simulink model "Pend_model"  (R2020b)
settings: Solver=VariableStepAuto  StartTime=0.0  StopTime=5  RelTol=1e-3
values from neighbouring files (symbols this model uses):
  A = eval(Ar)    [Script_pendul.m]    (also in extended_kalman_filter.m = I+Ts*eval(subs(jac,[x_sym,u_sym]',[x_est(:,k);u(:,k)])))
  B = eval(Br)    [Script_pendul.m]
  C = [1 0 0 0;0 0 1 0]    [Script_pendul.m]    (also in extended_kalman_filter.m = eval(subs(out_jac,x_sym',x_pred)))
  K = place(A,B,poles)    [Script_pendul.m]
  L = L'    [Script_pendul.m]
settings Model: Creator=tudor  LastModifiedBy=tudor

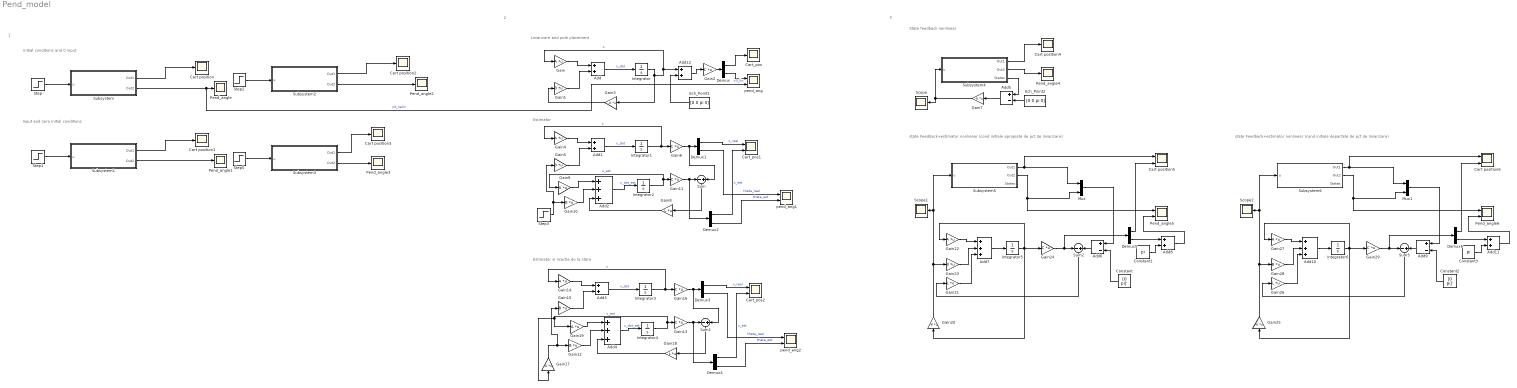
== system Pend_model ==
  note: 3
  note: State feedback nonlinear
  note: 2
  note: Estimator
  note: Liniarizare and pole placement
  note: 1
  note: Input and zero initial conditions
  note: Initial conditions and 0 input
  note: Estimator si reactie de la stare
  note: state Feedback+estimator nonlinear (cond initiale apropiate de pct de liniarizare)
  note: state Feedback+estimator nonlinear (cond initiale departate de pct de liniarizare)
  Add{,1,3,8,11..12} (6 alike) : Sum
  Add{2,4,7,10} (4 alike) : Sum  Inputs=+++
  Add5 : Sum  Inputs=+-
  Add6 : Sum  Inputs=+-
  Add9 : Sum  Inputs=+-
  Cart position{,1..4} (5 alike) : Scope
  Cart position5 : Scope  NumInputPorts=2
  Cart position6 : Scope  NumInputPorts=2
  Cart_pos : Scope
  Cart_pos1 : Scope  NumInputPorts=2
  Cart_pos2 : Scope  NumInputPorts=2
  Constant : Constant  Value=[0 pi]'
  Constant1 : Constant  Value=pi
  Constant2 : Constant  Value=[0 pi]'
  Constant3 : Constant  Value=pi
  Demux{,1..6} (7 alike) : Demux  Outputs=2
  Ech_Point1 : Constant  Value=[0 0 pi 0]
  Ech_Point2 : Constant  Value=[0 0 pi 0]
  Gain{,4,9,14,19,22,27} (7 alike) : Gain  Gain=A  Multiplication=Matrix(K*u)
  Gain{1,5,10,12,15,23,28} (7 alike) : Gain  Gain=B  Multiplication=Matrix(K*u)
  Gain{2,6,11,13,16,24,29} (7 alike) : Gain  Gain=C  Multiplication=Matrix(K*u)
  Gain{3,7,17,20,25} (5 alike) : Gain  Gain=-K  Multiplication=Matrix(K*u)
  Gain{8,18,21,26} (4 alike) : Gain  Gain=L  Multiplication=Matrix(K*u)
  Integrator : Integrator  InitialCondition=[0 0 0.01 0]
  Integrator1 : Integrator  InitialCondition=[0 0 0.1 0]
  Integrator2 : Integrator  InitialCondition=[0 0 0.5 0]
  Integrator3 : Integrator  InitialCondition=[0 0 0.1 0]
  Integrator4 : Integrator  InitialCondition=[0 0 1 0]
  Integrator5 : Integrator  InitialCondition=[0 0 0.5 0]
  Integrator6 : Integrator  InitialCondition=[0 0 0.5 0]
  Mux : Mux  Inputs=2
  Mux1 : Mux  Inputs=2
  Pend_angle{,1..4} (5 alike) : Scope
  Pend_angle5 : Scope  NumInputPorts=2
  Pend_angle6 : Scope  NumInputPorts=2
  Scope : Scope
  Scope1 : Scope
  Scope2 : Scope
  Step : Step  Time=0  After=0  SampleTime=0
  Step1 : Step  Before=10  After=0  SampleTime=0
  Step2 : Step  Time=0  After=0  SampleTime=0
  Step3 : Step  Time=0  After=0  SampleTime=0
  Step5 : Step  Before=0.1  After=0  SampleTime=0
  Subsystem : Subsystem
  Subsystem1 : Subsystem
  Subsystem2 : Subsystem
  Subsystem3 : Subsystem
  Subsystem4 : Subsystem
  Subsystem5 : Subsystem
  Subsystem6 : Subsystem
  Sum{,1..3} (4 alike) : Sum  Inputs=-|+
  pend_ang : Scope  NumInputPorts=2
  pend_ang1 : Scope  NumInputPorts=2
  pend_ang2 : Scope  NumInputPorts=2
  wires:
  Step/1 -> Subsystem/1(u)
  Subsystem/1(Out1) -> Cart position/1
  Subsystem/2(Out2) -> pend_ang/2, Pend_angle/1  "x3_nelin"
  Step1/1 -> Subsystem1/1(u)
  Subsystem1/2(Out2) -> Pend_angle1/1
  Subsystem1/1(Out1) -> Cart position1/1
  Step2/1 -> Subsystem2/1(u)
  Subsystem2/2(Out2) -> Pend_angle2/1
  Subsystem2/1(Out1) -> Cart position2/1
  Subsystem3/2(Out2) -> Pend_angle3/1
  Step5/1 -> Subsystem3/1(u)
  Subsystem3/1(Out1) -> Cart position3/1
  Gain/1 -> Add/1
  Gain1/1 -> Add/2
  Add/1 -> Integrator/1  "x_dot"
  Integrator/1 -> Gain3/1, Add12/1, Gain/1  "x"
  Gain3/1 -> Gain1/1
  Gain2/1 -> Demux/1
  Demux/1 -> Cart_pos/1
  Demux/2 -> pend_ang/1  "x3_lin"
  Gain6/1 -> Sum/2, Demux1/1
  Add1/1 -> Integrator1/1  "x_dot"
  Integrator1/1 -> Gain6/1, Gain4/1  "x"
  Gain5/1 -> Add1/2
  Demux1/2 -> pend_ang1/1  "theta_real"
  Gain4/1 -> Add1/1
  Demux1/1 -> Cart_pos1/1  "x_real"
  Sum/1 -> Gain8/1
  Gain8/1 -> Add2/3
  Add2/1 -> Integrator2/1  "x_dot_est"
  Integrator2/1 -> Gain9/1, Gain11/1  "x_est"
  Gain10/1 -> Add2/2
  Gain9/1 -> Add2/1
  Step3/1 -> Gain5/1, Gain10/1
  Gain11/1 -> Demux2/1, Sum/1
  Demux2/1 -> Cart_pos1/2  "x_est"
  Demux2/2 -> pend_ang1/2  "theta_est"
  Demux4/2 -> pend_ang2/2  "theta_est"
  Demux3/1 -> Cart_pos2/1  "x_real"
  Add3/1 -> Integrator3/1  "x_dot"
  Gain15/1 -> Add3/2
  Integrator3/1 -> Gain16/1, Gain14/1  "x"
  Gain16/1 -> Sum1/2, Demux3/1
  Gain13/1 -> Demux4/1, Sum1/1
  Integrator4/1 -> Gain17/1, Gain19/1, Gain13/1  "x_est"
  Demux3/2 -> pend_ang2/1  "theta_real"
  Gain17/1 -> Gain15/1, Gain12/1
  Demux4/1 -> Cart_pos2/2  "x_est"
  Gain18/1 -> Add4/3
  Sum1/1 -> Gain18/1
  Gain19/1 -> Add4/1
  Add4/1 -> Integrator4/1  "x_dot_est"
  Gain14/1 -> Add3/1
  Gain12/1 -> Add4/2
  Subsystem4/1(Out1) -> Cart position4/1
  Subsystem4/2(Out2) -> Pend_angle4/1
  Ech_Point2/1 -> Add5/2
  Gain7/1 -> Scope/1, Subsystem4/1(u)
  Subsystem4/3(States) -> Add5/1
  Add5/1 -> Gain7/1
  Subsystem5/2(Out2) -> Mux/2, Pend_angle5/1
  Subsystem5/1(Out1) -> Mux/1, Cart position5/1
  Sum2/1 -> Gain21/1
  Gain22/1 -> Add7/1
  Gain23/1 -> Add7/2
  Gain21/1 -> Add7/3
  Add7/1 -> Integrator5/1
  Demux5/1 -> Cart position5/2
  Gain24/1 -> Demux5/1, Sum2/1
  Integrator5/1 -> Gain22/1, Gain24/1, Gain20/1
  Gain20/1 -> Subsystem5/1(u), Scope1/1, Gain23/1
  Mux/1 -> Add6/1
  Add6/1 -> Sum2/2
  Constant/1 -> Add6/2
  Constant1/1 -> Add8/2
  Demux5/2 -> Add8/1
  Add8/1 -> Pend_angle5/2
  Subsystem6/2(Out2) -> Mux1/2, Pend_angle6/1
  Gain25/1 -> Subsystem6/1(u), Scope2/1, Gain28/1
  Subsystem6/1(Out1) -> Mux1/1, Cart position6/1
  Gain26/1 -> Add10/3
  Add10/1 -> Integrator6/1
  Integrator6/1 -> Gain27/1, Gain29/1, Gain25/1
  Demux6/1 -> Cart position6/2
  Gain28/1 -> Add10/2
  Constant3/1 -> Add11/2
  Sum3/1 -> Gain26/1
  Gain29/1 -> Demux6/1, Sum3/1
  Constant2/1 -> Add9/2
  Mux1/1 -> Add9/1
  Gain27/1 -> Add10/1
  Demux6/2 -> Add11/1
  Add9/1 -> Sum3/2
  Add11/1 -> Pend_angle6/2
  Ech_Point1/1 -> Add12/2
  Add12/1 -> Gain2/1

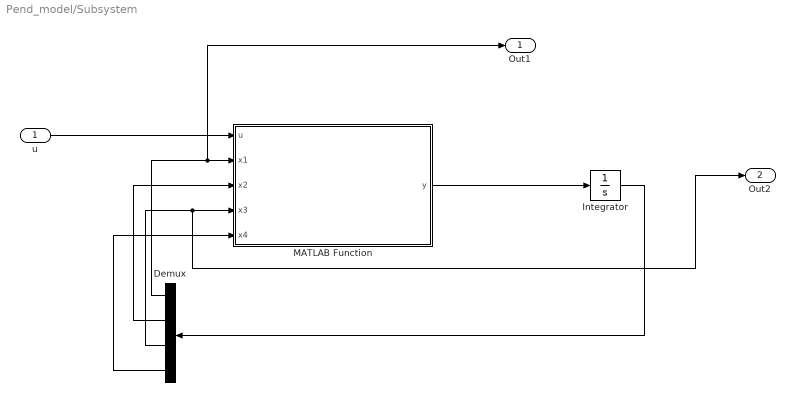
== system Pend_model/Subsystem ==
  u : Inport
  Demux : Demux
  Integrator : Integrator  InitialCondition=[0 0 pi+0.01 0]
  MATLAB Function : MATLAB Function  TreatAsAtomicUnit=on
  Out1 : Outport
  Out2 : Outport  Port=2
  wires:
  Integrator/1 -> Demux/1
  Demux/4 -> MATLAB Function/5(x4)
  MATLAB Function/1(y) -> Integrator/1
  Demux/3 -> Out2/1, MATLAB Function/4(x3)
  Demux/1 -> Out1/1, MATLAB Function/2(x1)
  Demux/2 -> MATLAB Function/3(x2)
  u/1 -> MATLAB Function/1(u)

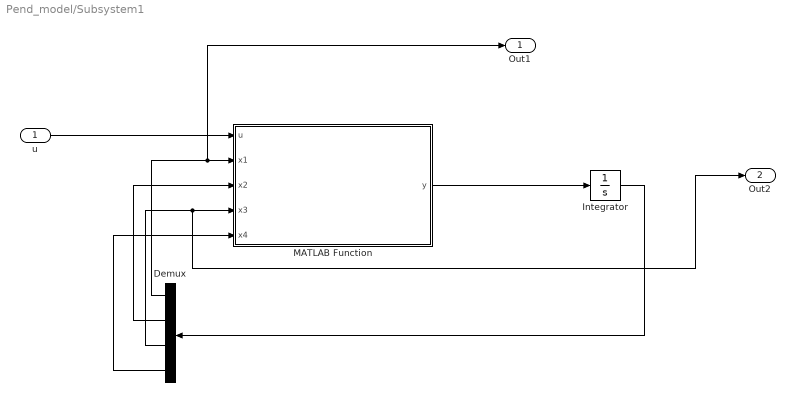
== system Pend_model/Subsystem1 ==
  u : Inport
  Demux : Demux
  Integrator : Integrator  InitialCondition=[0 0 0 0]
  MATLAB Function : MATLAB Function  TreatAsAtomicUnit=on
  Out1 : Outport
  Out2 : Outport  Port=2
  wires:
  Integrator/1 -> Demux/1
  Demux/4 -> MATLAB Function/5(x4)
  MATLAB Function/1(y) -> Integrator/1
  Demux/3 -> Out2/1, MATLAB Function/4(x3)
  Demux/1 -> Out1/1, MATLAB Function/2(x1)
  Demux/2 -> MATLAB Function/3(x2)
  u/1 -> MATLAB Function/1(u)

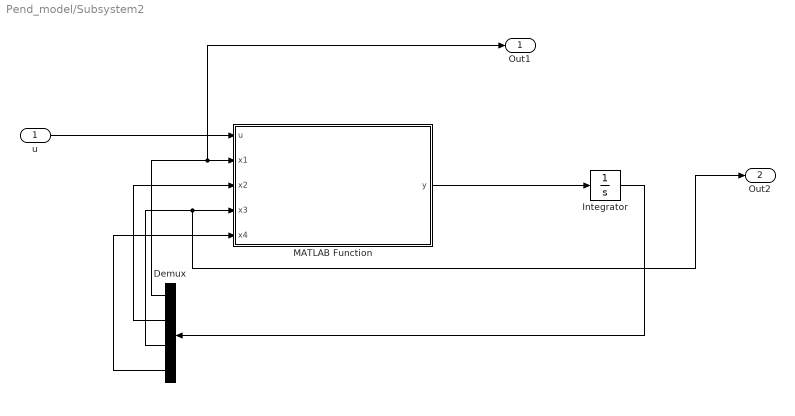
== system Pend_model/Subsystem2 ==
  u : Inport
  Demux : Demux
  Integrator : Integrator  InitialCondition=[0 0 pi 0]
  MATLAB Function : MATLAB Function  TreatAsAtomicUnit=on
  Out1 : Outport
  Out2 : Outport  Port=2
  wires:
  Integrator/1 -> Demux/1
  Demux/4 -> MATLAB Function/5(x4)
  MATLAB Function/1(y) -> Integrator/1
  Demux/3 -> Out2/1, MATLAB Function/4(x3)
  Demux/1 -> Out1/1, MATLAB Function/2(x1)
  Demux/2 -> MATLAB Function/3(x2)
  u/1 -> MATLAB Function/1(u)

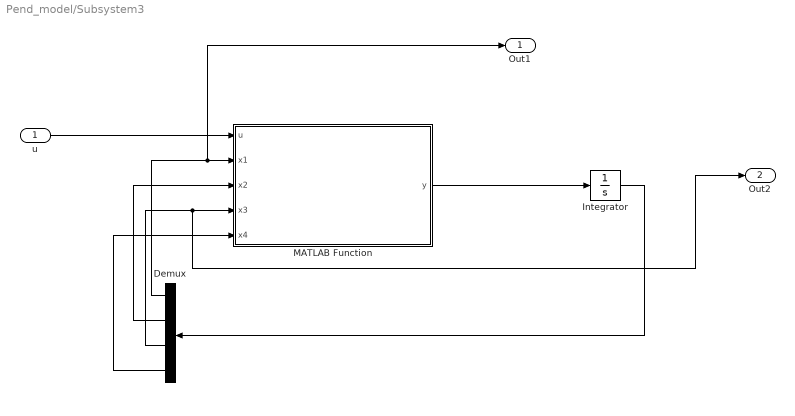
== system Pend_model/Subsystem3 ==
  u : Inport
  Demux : Demux
  Integrator : Integrator  InitialCondition=[0 0 0 0]
  MATLAB Function : MATLAB Function  TreatAsAtomicUnit=on
  Out1 : Outport
  Out2 : Outport  Port=2
  wires:
  Integrator/1 -> Demux/1
  Demux/4 -> MATLAB Function/5(x4)
  MATLAB Function/1(y) -> Integrator/1
  Demux/3 -> Out2/1, MATLAB Function/4(x3)
  Demux/1 -> Out1/1, MATLAB Function/2(x1)
  Demux/2 -> MATLAB Function/3(x2)
  u/1 -> MATLAB Function/1(u)

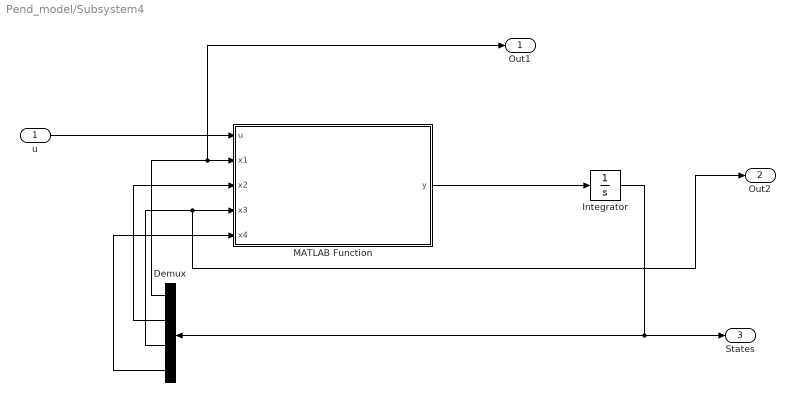
== system Pend_model/Subsystem4 ==
  u : Inport
  Demux : Demux
  Integrator : Integrator  InitialCondition=[0 0 pi+0.1 0]
  MATLAB Function : MATLAB Function  TreatAsAtomicUnit=on
  Out1 : Outport
  Out2 : Outport  Port=2
  States : Outport  Port=3
  wires:
  Integrator/1 -> States/1, Demux/1
  Demux/4 -> MATLAB Function/5(x4)
  MATLAB Function/1(y) -> Integrator/1
  Demux/3 -> Out2/1, MATLAB Function/4(x3)
  Demux/1 -> Out1/1, MATLAB Function/2(x1)
  Demux/2 -> MATLAB Function/3(x2)
  u/1 -> MATLAB Function/1(u)

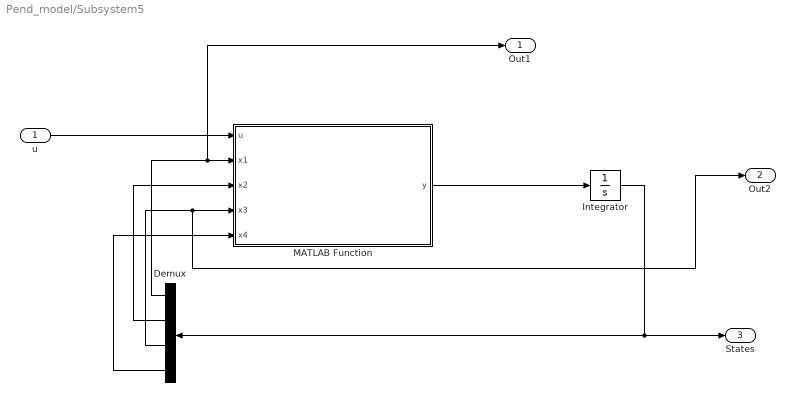
== system Pend_model/Subsystem5 ==
  u : Inport
  Demux : Demux
  Integrator : Integrator  InitialCondition=[0 0 pi+0.1 0]
  MATLAB Function : MATLAB Function  TreatAsAtomicUnit=on
  Out1 : Outport
  Out2 : Outport  Port=2
  States : Outport  Port=3
  wires:
  Integrator/1 -> States/1, Demux/1
  Demux/4 -> MATLAB Function/5(x4)
  MATLAB Function/1(y) -> Integrator/1
  Demux/3 -> Out2/1, MATLAB Function/4(x3)
  Demux/1 -> Out1/1, MATLAB Function/2(x1)
  Demux/2 -> MATLAB Function/3(x2)
  u/1 -> MATLAB Function/1(u)

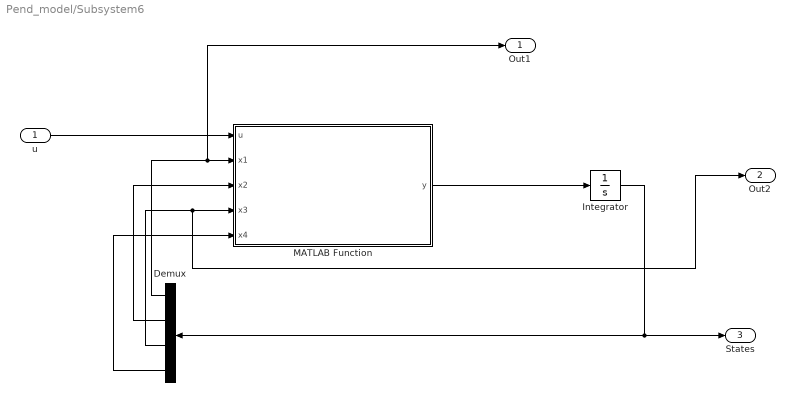
== system Pend_model/Subsystem6 ==
  u : Inport
  Demux : Demux
  Integrator : Integrator  InitialCondition=[0 0 pi+1 0]
  MATLAB Function : MATLAB Function  TreatAsAtomicUnit=on
  Out1 : Outport
  Out2 : Outport  Port=2
  States : Outport  Port=3
  wires:
  Integrator/1 -> States/1, Demux/1
  Demux/4 -> MATLAB Function/5(x4)
  MATLAB Function/1(y) -> Integrator/1
  Demux/3 -> Out2/1, MATLAB Function/4(x3)
  Demux/1 -> Out1/1, MATLAB Function/2(x1)
  Demux/2 -> MATLAB Function/3(x2)
  u/1 -> MATLAB Function/1(u)

== matlab function Pend_model/Subsystem1/MATLAB Function ==
  data: u input; y output; x1 input; x2 input; x3 input; x4 input
function y = cart_pendulum(u,x1,x2,x3,x4)
M=0.5;
m=0.5;
b=0.1;
l=0.3;
I=0.006;
g=9.8;

c1=M+m-m^2*l^2*cos(x3)^2/(I+m*l^2)
c2=-m*l/(I+m*l^2)*cos(x3)/(m+M-m^2*l^2/(I+m*l^2)*cos(x3)^2)

dx1=x2
dx2=1/c1*(-b*x2+m^2*l^2*g/(I+m*l^2)*sin(2*x3)/2+m*l*x4^2*sin(x3)+u)
dx3=x4
dx4=c2*(-b*x2+m^2*l^2*g/2/(I+m*l^2)*sin(2*x3)+m*l*x4^2*sin(x3)+u)-m*g*l/(I+m*l^2)*sin(x3)

y = [dx1 dx2 dx3 dx4];

== matlab function Pend_model/Subsystem/MATLAB Function ==
  data: u input; y output; x1 input; x2 input; x3 input; x4 input
function y = cart_pendulum(u,x1,x2,x3,x4)
M=0.5;
m=0.5;
b=0.1;
l=0.3;
I=0.006;
g=9.8;

c1=M+m-m^2*l^2*cos(x3)^2/(I+m*l^2)
c2=-m*l/(I+m*l^2)*cos(x3)/(m+M-m^2*l^2/(I+m*l^2)*cos(x3)^2)

dx1=x2
dx2=1/c1*(-b*x2+m^2*l^2*g/(I+m*l^2)*sin(2*x3)/2+m*l*x4^2*sin(x3)+u)
dx3=x4
dx4=c2*(-b*x2+m^2*l^2*g/2/(I+m*l^2)*sin(2*x3)+m*l*x4^2*sin(x3)+u)-m*g*l/(I+m*l^2)*sin(x3)

y = [dx1 dx2 dx3 dx4];

== matlab function Pend_model/Subsystem2/MATLAB Function ==
  data: u input; y output; x1 input; x2 input; x3 input; x4 input
function y = cart_pendulum(u,x1,x2,x3,x4)
M=0.5;
m=0.5;
b=0.1;
l=0.3;
I=0.006;
g=9.8;

c1=M+m-m^2*l^2*cos(x3)^2/(I+m*l^2)
c2=-m*l/(I+m*l^2)*cos(x3)/(m+M-m^2*l^2/(I+m*l^2)*cos(x3)^2)

dx1=x2
dx2=1/c1*(-b*x2+m^2*l^2*g/(I+m*l^2)*sin(2*x3)/2+m*l*x4^2*sin(x3)+u)
dx3=x4
dx4=c2*(-b*x2+m^2*l^2*g/2/(I+m*l^2)*sin(2*x3)+m*l*x4^2*sin(x3)+u)-m*g*l/(I+m*l^2)*sin(x3)

y = [dx1 dx2 dx3 dx4];

== matlab function Pend_model/Subsystem3/MATLAB Function ==
  data: u input; y output; x1 input; x2 input; x3 input; x4 input
function y = cart_pendulum(u,x1,x2,x3,x4)
M=0.5;
m=0.5;
b=0.1;
l=0.3;
I=0.006;
g=9.8;

c1=M+m-m^2*l^2*cos(x3)^2/(I+m*l^2)
c2=-m*l/(I+m*l^2)*cos(x3)/(m+M-m^2*l^2/(I+m*l^2)*cos(x3)^2)

dx1=x2
dx2=1/c1*(-b*x2+m^2*l^2*g/(I+m*l^2)*sin(2*x3)/2+m*l*x4^2*sin(x3)+u)
dx3=x4
dx4=c2*(-b*x2+m^2*l^2*g/2/(I+m*l^2)*sin(2*x3)+m*l*x4^2*sin(x3)+u)-m*g*l/(I+m*l^2)*sin(x3)

y = [dx1 dx2 dx3 dx4];

== matlab function Pend_model/Subsystem4/MATLAB Function ==
  data: u input; y output; x1 input; x2 input; x3 input; x4 input
function y = cart_pendulum(u,x1,x2,x3,x4)
M=0.5;
m=0.5;
b=0.1;
l=0.3;
I=0.006;
g=9.8;

c1=M+m-m^2*l^2*cos(x3)^2/(I+m*l^2)
c2=-m*l/(I+m*l^2)*cos(x3)/(m+M-m^2*l^2/(I+m*l^2)*cos(x3)^2)

dx1=x2
dx2=1/c1*(-b*x2+m^2*l^2*g/(I+m*l^2)*sin(2*x3)/2+m*l*x4^2*sin(x3)+u)
dx3=x4
dx4=c2*(-b*x2+m^2*l^2*g/2/(I+m*l^2)*sin(2*x3)+m*l*x4^2*sin(x3)+u)-m*g*l/(I+m*l^2)*sin(x3)

y = [dx1 dx2 dx3 dx4];

== matlab function Pend_model/Subsystem5/MATLAB Function ==
  data: u input; y output; x1 input; x2 input; x3 input; x4 input
function y = cart_pendulum(u,x1,x2,x3,x4)
M=0.5;
m=0.5;
b=0.1;
l=0.3;
I=0.006;
g=9.8;

c1=M+m-m^2*l^2*cos(x3)^2/(I+m*l^2)
c2=-m*l/(I+m*l^2)*cos(x3)/(m+M-m^2*l^2/(I+m*l^2)*cos(x3)^2)

dx1=x2
dx2=1/c1*(-b*x2+m^2*l^2*g/(I+m*l^2)*sin(2*x3)/2+m*l*x4^2*sin(x3)+u)
dx3=x4
dx4=c2*(-b*x2+m^2*l^2*g/2/(I+m*l^2)*sin(2*x3)+m*l*x4^2*sin(x3)+u)-m*g*l/(I+m*l^2)*sin(x3)

y = [dx1 dx2 dx3 dx4];

== matlab function Pend_model/Subsystem6/MATLAB Function ==
  data: u input; y output; x1 input; x2 input; x3 input; x4 input
function y = cart_pendulum(u,x1,x2,x3,x4)
M=0.5;
m=0.5;
b=0.1;
l=0.3;
I=0.006;
g=9.8;

c1=M+m-m^2*l^2*cos(x3)^2/(I+m*l^2)
c2=-m*l/(I+m*l^2)*cos(x3)/(m+M-m^2*l^2/(I+m*l^2)*cos(x3)^2)

dx1=x2
dx2=1/c1*(-b*x2+m^2*l^2*g/(I+m*l^2)*sin(2*x3)/2+m*l*x4^2*sin(x3)+u)
dx3=x4
dx4=c2*(-b*x2+m^2*l^2*g/2/(I+m*l^2)*sin(2*x3)+m*l*x4^2*sin(x3)+u)-m*g*l/(I+m*l^2)*sin(x3)

y = [dx1 dx2 dx3 dx4];
